simulink model "am_2"  (R2018a)
settings: Solver=VariableStepAuto  StartTime=0.0  StopTime=10.0  MaxStep=0.001  RelTol=1e-3
undefined symbols (not defined in the file or in its folder): magnitude
libraries: commanapbnd3 x1, dspstat3 x1, commrandsrc3 x1
settings Model: Creator=sdf  LastModifiedBy=sdf

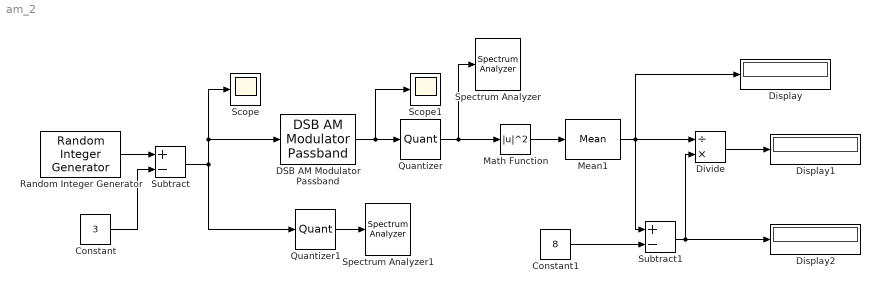
== system am_2 ==
  Constant : Constant  Value=3
  Constant1 : Constant  Value=8
  DSB AM Modulator Passband : commanapbnd3/DSB AM Modulator Passband  Fc=100  Ph=0  Offset=4
      settings: SourceProductName=Communications System Toolbox  SourceProductBaseCode=CM
  Display : Display
  Display1 : Display
  Display2 : Display
  Divide : Product  Inputs=/*
  Math Function : Math  Operator=magnitude^2  SaturateOnIntegerOverflow=on
  Mean1 : dspstat3/Mean  run=on  InputProcessing=Columns as channels (frame based)  reset_popup=None  directionMode=Each column  dimension=1  roiEnable=off  roiType=Rectangles  roiPortion=Entire ROI  roiOutput=Individual statistics for each ROI  roiFlag=off  roundingMode=Floor  overflowMode=off  outputDataTypeStr=Inherit: Same as accumulator  outputMin=[]  outputMax=[]  outputLastDataTypeStr=Inherit: Same as accumulator
  Quantizer : Quantizer  QuantizationInterval=0.001  LinearizeAsGain=off
  Quantizer1 : Quantizer  QuantizationInterval=0.001  LinearizeAsGain=off
  Random Integer Generator : commrandsrc3/Random Integer Generator  SetSize=7  SeedSource=Parameter  Seed=1234  SampleTime=1/10  SamplesPerFrame=10  OutputDataType=double  SimulateUsing=Interpreted execution
  Scope : Scope
  Scope1 : Scope
  Spectrum Analyzer : SpectrumAnalyzer
  Spectrum Analyzer1 : SpectrumAnalyzer
  Subtract : Sum  Inputs=+-
  Subtract1 : Sum  Inputs=+-
  wires:
  Random Integer Generator/1 -> Subtract/1
  Constant/1 -> Subtract/2
  Subtract/1 -> Scope/1, DSB AM Modulator Passband/1, Quantizer1/1
  DSB AM Modulator Passband/1 -> Scope1/1, Quantizer/1
  Quantizer1/1 -> Spectrum Analyzer1/1
  Quantizer/1 -> Math Function/1, Spectrum Analyzer/1
  Math Function/1 -> Mean1/1
  Mean1/1 -> Display/1, Subtract1/1, Divide/1
  Subtract1/1 -> Display2/1, Divide/2
  Constant1/1 -> Subtract1/2
  Divide/1 -> Display1/1
